simulink model "RTR_IK"  (R2020a)
settings: Solver=ode45  StartTime=0.0  StopTime=T  RelTol=1e-8
values from neighbouring files (symbols this model uses):
  g = 9.81    [TestingIkRTR.m]    (also in TestingScript.m; TestingScriptRTR.m)
  Kd1 = Kp1/10    (= 100)    [TestingIkRTR.m]    (also in TestingScript.m; TestingScriptRTR.m)
  Kp1 = 1000    [TestingIkRTR.m]    (also in TestingScript.m; TestingScriptRTR.m)
  l2 = 0.3    [TestingIkRTR.m]    (also in TestingScriptRTR.m)
  l3 = 0.2    [TestingIkRTR.m]    (also in TestingScriptRTR.m)
  m2 = 20    [TestingIkRTR.m]    (also in TestingScriptRTR.m)
  m3 = 20    [TestingIkRTR.m]    (also in TestingScriptRTR.m)
settings Model: Creator=ja  LastModifiedBy=ja

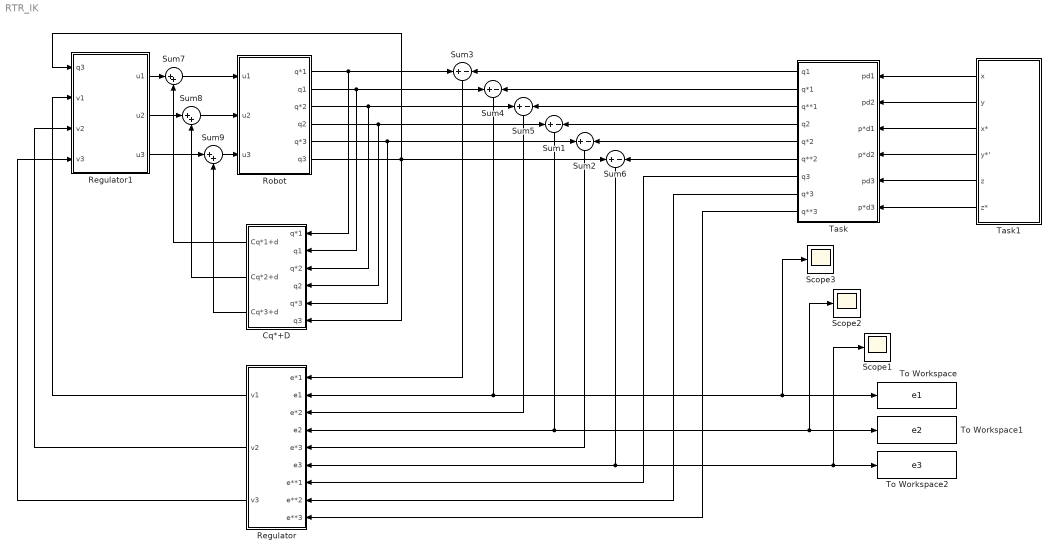
== system RTR_IK ==
  Cq*+D : Subsystem
  Regulator : Subsystem
  Regulator1 : Subsystem
  Robot : Subsystem
  Scope1 : Scope
  Scope2 : Scope
  Scope3 : Scope
  Sum{1..6} (6 alike) : Sum  Inputs=+-
  Sum7 : Sum  Inputs=|++
  Sum8 : Sum  Inputs=|++
  Sum9 : Sum  Inputs=|++
  Task : Subsystem
  Task1 : Subsystem
  To Workspace : ToWorkspace  VariableName=e1  SampleTime=-1
  To Workspace1 : ToWorkspace  VariableName=e2  SampleTime=-1
  To Workspace2 : ToWorkspace  VariableName=e3  SampleTime=-1
  wires:
  Robot/1(q*1) -> Cq*+D/1(q*1), Sum3/1
  Task/1(q1) -> Sum3/2
  Robot/2(q1) -> Cq*+D/2(q1), Sum4/1
  Task/2(q*1) -> Sum4/2
  Task/3(q**1) -> Sum5/2
  Robot/3(q*2) -> Cq*+D/3(q*2), Sum5/1
  Task/4(q2) -> Sum1/2
  Robot/4(q2) -> Cq*+D/4(q2), Sum1/1
  Task/5(q*2) -> Sum2/2
  Robot/5(q*3) -> Cq*+D/5(q*3), Sum2/1
  Task/6(q**2) -> Sum6/2
  Robot/6(q3) -> Regulator1/1(q3), Cq*+D/6(q3), Sum6/1
  Sum3/1 -> Regulator/1(e*1)
  Sum4/1 -> Scope3/1, To Workspace/1, Regulator/2(e1)
  Sum5/1 -> Regulator/3(e*2)
  Sum1/1 -> Scope2/1, To Workspace1/1, Regulator/4(e2)
  Sum2/1 -> Regulator/5(e*3)
  Sum6/1 -> Scope1/1, To Workspace2/1, Regulator/6(e3)
  Regulator/1(" v1") -> Regulator1/2(v1)
  Regulator/2(v2) -> Regulator1/3(v2)
  Regulator/3(v3) -> Regulator1/4(v3)
  Sum7/1 -> Robot/1(u1)
  Regulator1/1(" u1") -> Sum7/1
  Regulator1/2(u2) -> Sum8/1
  Sum8/1 -> Robot/2(u2)
  Regulator1/3(u3) -> Sum9/1
  Sum9/1 -> Robot/3(u3)
  Cq*+D/1(" Cq*1+d") -> Sum7/2
  Cq*+D/2(Cq*2+d) -> Sum8/2
  Cq*+D/3(Cq*3+d) -> Sum9/2
  Task/7(q3) -> Regulator/7(e**1)
  Task/8(q*3) -> Regulator/8(e**2)
  Task/9(q**3) -> Regulator/9(e**3)
  Task1/6(z*) -> Task/6(p*d3)
  Task1/5(z) -> Task/5(pd3)
  Task1/4(y*') -> Task/4(p*d2)
  Task1/1(x) -> Task/1(pd1)
  Task1/2(y) -> Task/2(pd2)
  Task1/3(x*) -> Task/3(p*d1)

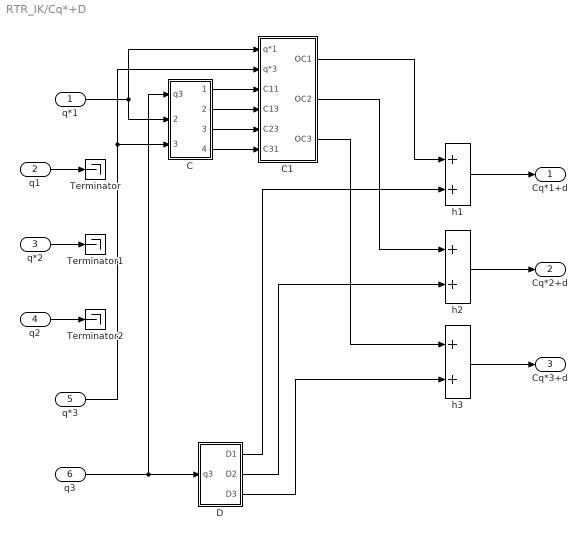
== system RTR_IK/Cq*+D ==
  q*1 : Inport
  q1 : Inport  Port=2
  q*2 : Inport  Port=3
  q2 : Inport  Port=4
  q*3 : Inport  Port=5
  q3 : Inport  Port=6
  C : Subsystem
  C1 : Subsystem
  D : Subsystem
  Terminator : Terminator
  Terminator1 : Terminator
  Terminator2 : Terminator
  h1 : Sum
  h2 : Sum
  h3 : Sum
  " Cq*1+d" : Outport
  Cq*2+d : Outport  Port=2
  Cq*3+d : Outport  Port=3
  wires:
  D/1(D1) -> h1/2
  D/2(D2) -> h2/2
  C1/2(OC2) -> h2/1
  D/3(D3) -> h3/2
  C/2(C13) -> C1/4(C13)
  C/1(C11) -> C1/3(C11)
  C/3(C23) -> C1/5(C23)
  C1/1(OC1) -> h1/1
  C/4(C31) -> C1/6(C31)
  C1/3(OC3) -> h3/1
  q3/1 -> C/1(q3), D/1(q3)
  h1/1 -> " Cq*1+d"/1
  h2/1 -> Cq*2+d/1
  h3/1 -> Cq*3+d/1
  q*1/1 -> C1/1(q*1), C/2(q*1)
  q*3/1 -> C/3(q*3), C1/2(q*3)
  q1/1 -> Terminator/1
  q*2/1 -> Terminator1/1
  q2/1 -> Terminator2/1

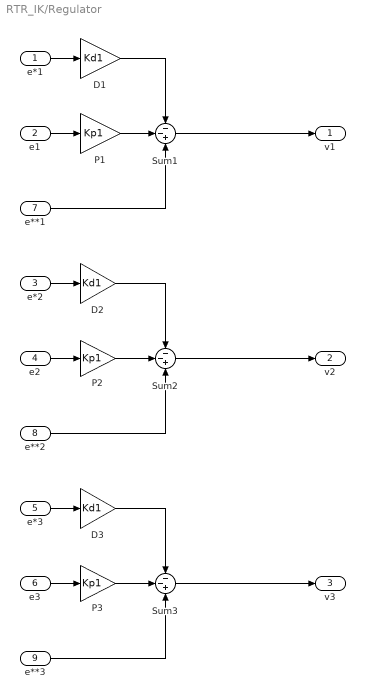
== system RTR_IK/Regulator ==
  e*1 : Inport
  e1 : Inport  Port=2
  e*2 : Inport  Port=3
  e2 : Inport  Port=4
  e*3 : Inport  Port=5
  e3 : Inport  Port=6
  e**1 : Inport  Port=7
  e**2 : Inport  Port=8
  e**3 : Inport  Port=9
  D1 : Gain  Gain=Kd1
  D2 : Gain  Gain=Kd1
  D3 : Gain  Gain=Kd1
  P1 : Gain  Gain=Kp1
  P2 : Gain  Gain=Kp1
  P3 : Gain  Gain=Kp1
  Sum1 : Sum  Inputs=--+
  Sum2 : Sum  Inputs=--+
  Sum3 : Sum  Inputs=--+
  " v1" : Outport
  v2 : Outport  Port=2
  v3 : Outport  Port=3
  wires:
  e2/1 -> P2/1
  Sum2/1 -> v2/1
  e*2/1 -> D2/1
  e1/1 -> P1/1
  Sum1/1 -> " v1"/1
  e*1/1 -> D1/1
  D1/1 -> Sum1/1
  P1/1 -> Sum1/2
  D2/1 -> Sum2/1
  P2/1 -> Sum2/2
  e*3/1 -> D3/1
  Sum3/1 -> v3/1
  P3/1 -> Sum3/2
  D3/1 -> Sum3/1
  e3/1 -> P3/1
  e**1/1 -> Sum1/3
  e**2/1 -> Sum2/3
  e**3/1 -> Sum3/3

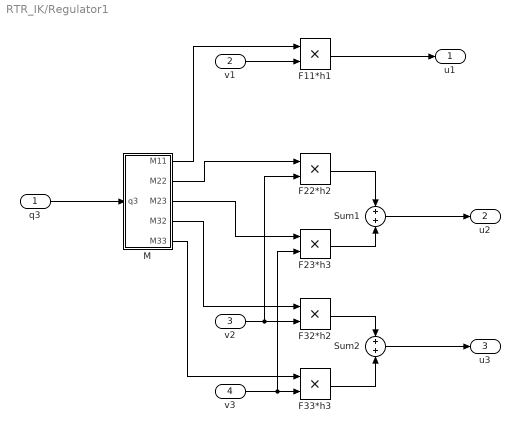
== system RTR_IK/Regulator1 ==
  q3 : Inport
  v1 : Inport  Port=2
  v2 : Inport  Port=3
  v3 : Inport  Port=4
  F11*h1 : Product
  F22*h2 : Product
  F23*h3 : Product
  F32*h2 : Product
  F33*h3 : Product
  M : Subsystem
  Sum1 : Sum
  Sum2 : Sum
  " u1" : Outport
  u2 : Outport  Port=2
  u3 : Outport  Port=3
  wires:
  q3/1 -> M/1(q3)
  F23*h3/1 -> Sum1/2
  F33*h3/1 -> Sum2/2
  F22*h2/1 -> Sum1/1
  F32*h2/1 -> Sum2/1
  v3/1 -> F23*h3/2, F33*h3/2
  v2/1 -> F22*h2/2, F32*h2/2
  v1/1 -> F11*h1/2
  M/1(M11) -> F11*h1/1
  M/2(M22) -> F22*h2/1
  M/3(M23) -> F23*h3/1
  M/4(M32) -> F32*h2/1
  M/5(M33) -> F33*h3/1
  F11*h1/1 -> " u1"/1
  Sum1/1 -> u2/1
  Sum2/1 -> u3/1

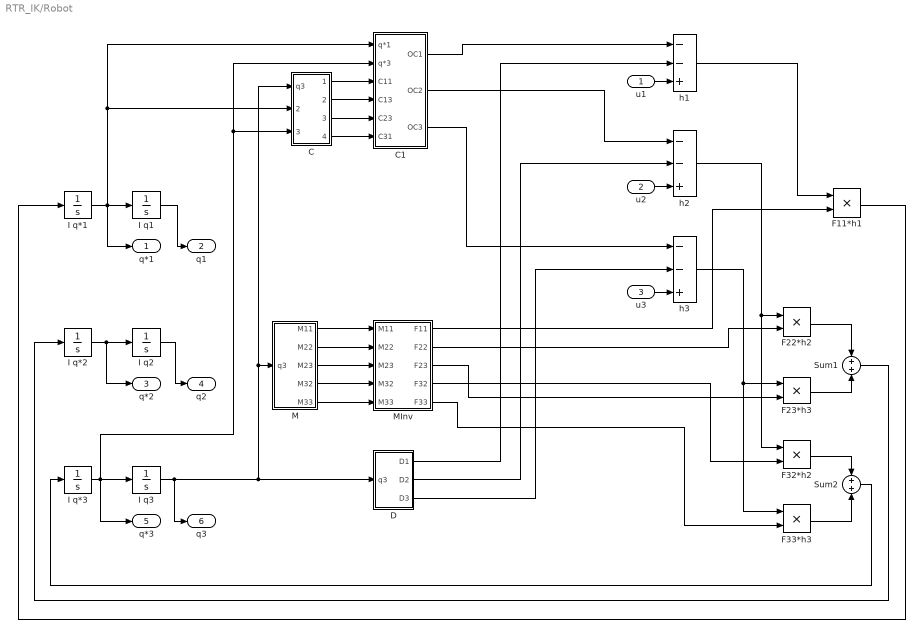
== system RTR_IK/Robot ==
  u1 : Inport
  u2 : Inport  Port=2
  u3 : Inport  Port=3
  C : Subsystem
  C1 : Subsystem
  D : Subsystem
  F11*h1 : Product
  F22*h2 : Product
  F23*h3 : Product
  F32*h2 : Product
  F33*h3 : Product
  I q*1 : Integrator
  I q*2 : Integrator
  I q*3 : Integrator
  I q1 : Integrator
  I q2 : Integrator
  I q3 : Integrator
  M : Subsystem
  MInv : MATLAB Function  TreatAsAtomicUnit=on
  Sum1 : Sum
  Sum2 : Sum
  h1 : Sum  Inputs=--+
  h2 : Sum  Inputs=--+
  h3 : Sum  Inputs=--+
  q*1 : Outport
  q1 : Outport  Port=2
  q*2 : Outport  Port=3
  q2 : Outport  Port=4
  q*3 : Outport  Port=5
  q3 : Outport  Port=6
  wires:
  I q2/1 -> q2/1
  F11*h1/1 -> I q*1/1
  I q*1/1 -> q*1/1, C1/1(q*1), C/2(q*1), I q1/1
  Sum1/1 -> I q*2/1
  I q1/1 -> q1/1
  F23*h3/1 -> Sum1/2
  I q*2/1 -> q*2/1, I q2/1
  F22*h2/1 -> Sum1/1
  u2/1 -> h2/3
  C/1(C11) -> C1/3(C11)
  C/2(C13) -> C1/4(C13)
  C/3(C23) -> C1/5(C23)
  C/4(C31) -> C1/6(C31)
  C1/1(OC1) -> h1/1
  F32*h2/1 -> Sum2/1
  F33*h3/1 -> Sum2/2
  Sum2/1 -> I q*3/1
  I q*3/1 -> C1/2(q*3), C/3(q*3), I q3/1, q*3/1
  I q3/1 -> q3/1, C/1(q3), M/1(q3), D/1(q3)
  u3/1 -> h3/3
  D/3(D3) -> h3/2
  D/2(D2) -> h2/2
  C1/2(OC2) -> h2/1
  C1/3(OC3) -> h3/1
  h2/1 -> F32*h2/1, F22*h2/1
  h3/1 -> F33*h3/1, F23*h3/1
  MInv/2(F22) -> F22*h2/2
  MInv/3(F23) -> F23*h3/2
  MInv/4(F32) -> F32*h2/2
  MInv/5(F33) -> F33*h3/2
  h1/1 -> F11*h1/1
  MInv/1(F11) -> F11*h1/2
  u1/1 -> h1/3
  D/1(D1) -> h1/2
  M/1(M11) -> MInv/1(M11)
  M/2(M22) -> MInv/2(M22)
  M/3(M23) -> MInv/3(M23)
  M/4(M32) -> MInv/4(M32)
  M/5(M33) -> MInv/5(M33)

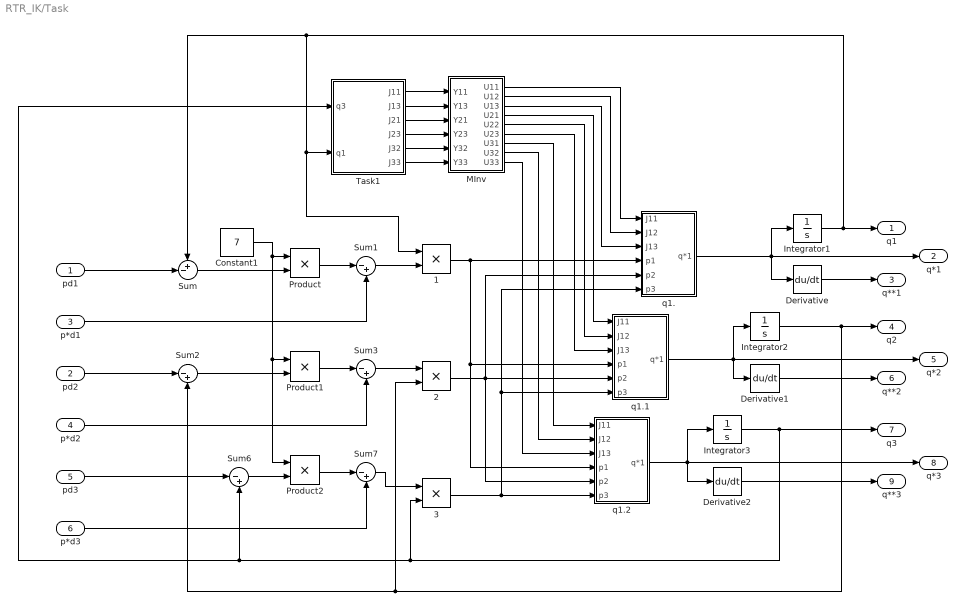
== system RTR_IK/Task ==
  pd1 : Inport
  pd2 : Inport  Port=2
  p*d1 : Inport  Port=3
  p*d2 : Inport  Port=4
  pd3 : Inport  Port=5
  p*d3 : Inport  Port=6
  1 : Product
  2 : Product
  3 : Product
  Constant1 : Constant  Value=7
  Derivative : Derivative
  Derivative1 : Derivative
  Derivative2 : Derivative
  Integrator1 : Integrator
  Integrator2 : Integrator
  Integrator3 : Integrator  InitialCondition=0.1
  MInv : MATLAB Function  TreatAsAtomicUnit=on
  Product : Product
  Product1 : Product
  Product2 : Product
  Sum : Sum  Inputs=+-|
  Sum{1..3,6..7} (5 alike) : Sum  Inputs=|-+
  Task1 : Subsystem
  q1. : Subsystem
  q1.1 : Subsystem
  q1.2 : Subsystem
  q1 : Outport
  q*1 : Outport  Port=2
  q**1 : Outport  Port=3
  q2 : Outport  Port=4
  q*2 : Outport  Port=5
  q**2 : Outport  Port=6
  q3 : Outport  Port=7
  q*3 : Outport  Port=8
  q**3 : Outport  Port=9
  wires:
  pd1/1 -> Sum/2
  Sum1/1 -> 1/2
  Product/1 -> Sum1/1
  Product1/1 -> Sum3/1
  Sum/1 -> Product/2
  Integrator1/1 -> q1/1, Sum/1, 1/1, Task1/2(q1)
  p*d2/1 -> Sum3/2
  Sum2/1 -> Product1/2
  Integrator2/1 -> q2/1, Sum2/2, 2/2
  pd2/1 -> Sum2/1
  p*d1/1 -> Sum1/2
  Sum3/1 -> 2/1
  Sum6/1 -> Product2/2
  pd3/1 -> Sum6/1
  Constant1/1 -> Product2/1, Product1/1, Product/1
  p*d3/1 -> Sum7/2
  Product2/1 -> Sum7/1
  Sum7/1 -> 3/1
  Task1/1(J11) -> MInv/1(Y11)
  Task1/2(J13) -> MInv/2(Y13)
  Task1/3(J21) -> MInv/3(Y21)
  Task1/4(J23) -> MInv/4(Y23)
  Task1/5(J32) -> MInv/5(Y32)
  Task1/6(J33) -> MInv/6(Y33)
  1/1 -> q1./4(p1), q1.2/4(p1), q1.1/4(p1)
  2/1 -> q1.2/5(p2), q1.1/5(p2), q1./5(p2)
  3/1 -> q1./6(p3), q1.1/6(p3), q1.2/6(p3)
  MInv/1(U11) -> q1./1(J11)
  MInv/2(U12) -> q1./2(J12)
  MInv/3(U13) -> q1./3(J13)
  MInv/4(U21) -> q1.1/1(J11)
  MInv/5(U22) -> q1.1/2(J12)
  MInv/6(U23) -> q1.1/3(J13)
  MInv/7(U31) -> q1.2/1(J11)
  MInv/8(U32) -> q1.2/2(J12)
  MInv/9(U33) -> q1.2/3(J13)
  Integrator3/1 -> q3/1, 3/2, Task1/1(q3), Sum6/2
  Derivative/1 -> q**1/1
  q1./1(q*1) -> Derivative/1, Integrator1/1, q*1/1
  q1.1/1(q*1) -> Derivative1/1, Integrator2/1, q*2/1
  q1.2/1(q*1) -> Integrator3/1, Derivative2/1, q*3/1
  Derivative1/1 -> q**2/1
  Derivative2/1 -> q**3/1

== system RTR_IK/Task1 ==
  Clock1 : Clock
  Fcn6 : Fcn  Expr=2*cos(2*u)
  Fcn7 : Fcn  Expr=0.1
  Fcn8 : Fcn  Expr=0.1+u
  Fcn9 : Fcn  Expr=-2*sin(2*u)
  Integrator8 : Integrator
  Integrator9 : Integrator  InitialCondition=1
  x : Outport
  y : Outport  Port=2
  x* : Outport  Port=3
  y*' : Outport  Port=4
  z : Outport  Port=5
  z* : Outport  Port=6
  wires:
  Fcn8/1 -> z/1
  Fcn7/1 -> z*/1
  Integrator8/1 -> x/1
  Fcn6/1 -> x*/1, Integrator8/1
  Clock1/1 -> Fcn8/1, Fcn7/1, Fcn6/1, Fcn9/1
  Integrator9/1 -> y/1
  Fcn9/1 -> y*'/1, Integrator9/1

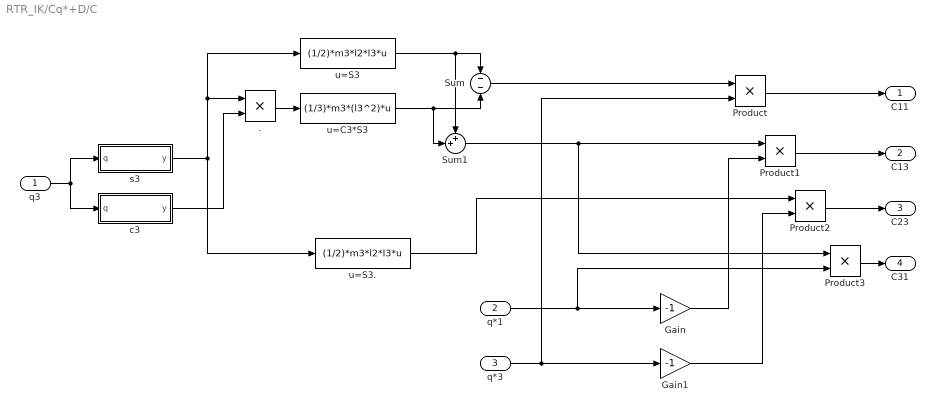
== system RTR_IK/Cq*+D/C ==
  q3 : Inport
  q*1 : Inport  Port=2
  q*3 : Inport  Port=3
  . : Product
  Gain : Gain  Gain=-1
  Gain1 : Gain  Gain=-1
  Product{,1..3} (4 alike) : Product
  Sum : Sum  Inputs=--
  Sum1 : Sum  Inputs=++|
  c3 : MATLAB Function  TreatAsAtomicUnit=on
  s3 : MATLAB Function  TreatAsAtomicUnit=on
  u=C3*S3 : Fcn  Expr=(1/3)*m3*(l3^2)*u
  u=S3 : Fcn  Expr=(1/2)*m3*l2*l3*u
  u=S3. : Fcn  Expr=(1/2)*m3*l2*l3*u
  C11 : Outport
  C13 : Outport  Port=2
  C23 : Outport  Port=3
  C31 : Outport  Port=4
  wires:
  q3/1 -> s3/1(q), c3/1(q)
  c3/1(y) -> ./2
  s3/1(y) -> u=S3./1, ./1, u=S3/1
  ./1 -> u=C3*S3/1
  u=C3*S3/1 -> Sum1/2, Sum/2
  u=S3/1 -> Sum1/1, Sum/1
  Gain1/1 -> Product2/2
  Product/1 -> C11/1
  Product2/1 -> C23/1
  Product1/1 -> C13/1
  Sum/1 -> Product/1
  q*1/1 -> Gain/1, Product3/2
  q*3/1 -> Gain1/1, Product/2
  Product3/1 -> C31/1
  Gain/1 -> Product1/2
  Sum1/1 -> Product1/1, Product3/1
  u=S3./1 -> Product2/1

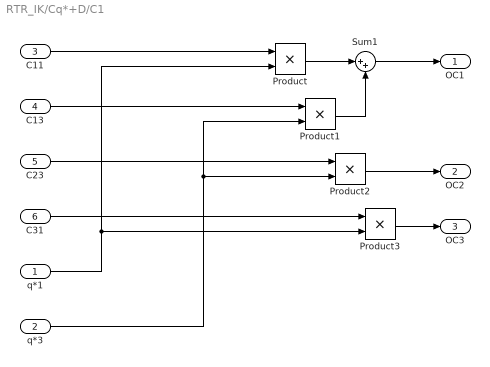
== system RTR_IK/Cq*+D/C1 ==
  q*1 : Inport
  q*3 : Inport  Port=2
  C11 : Inport  Port=3
  C13 : Inport  Port=4
  C23 : Inport  Port=5
  C31 : Inport  Port=6
  Product{,1..3} (4 alike) : Product
  Sum1 : Sum  Inputs=|++
  OC1 : Outport
  OC2 : Outport  Port=2
  OC3 : Outport  Port=3
  wires:
  C11/1 -> Product/1
  C13/1 -> Product1/1
  C23/1 -> Product2/1
  C31/1 -> Product3/1
  Product3/1 -> OC3/1
  Product2/1 -> OC2/1
  q*1/1 -> Product3/2, Product/2
  q*3/1 -> Product2/2, Product1/2
  Product/1 -> Sum1/1
  Sum1/1 -> OC1/1
  Product1/1 -> Sum1/2

== system RTR_IK/Cq*+D/D ==
  q3 : Inport
  . : Fcn  Expr=1/2*m3*l3*u
  Constant : Constant  Value=g
  Constant1 : Constant  Value=m3
  Constant2 : Constant  Value=m2
  Constant3 : Constant  Value=0
  Product : Product
  Product1 : Product
  Sum : Sum
  c3 : MATLAB Function  TreatAsAtomicUnit=on
  D1 : Outport
  D2 : Outport  Port=2
  D3 : Outport  Port=3
  wires:
  c3/1(y) -> ./1
  Sum/1 -> Product/1
  Constant/1 -> Product/2, Product1/1
  ./1 -> Product1/2
  Constant2/1 -> Sum/2
  Constant1/1 -> Sum/1
  q3/1 -> c3/1(q)
  Product/1 -> D2/1
  Product1/1 -> D3/1
  Constant3/1 -> D1/1

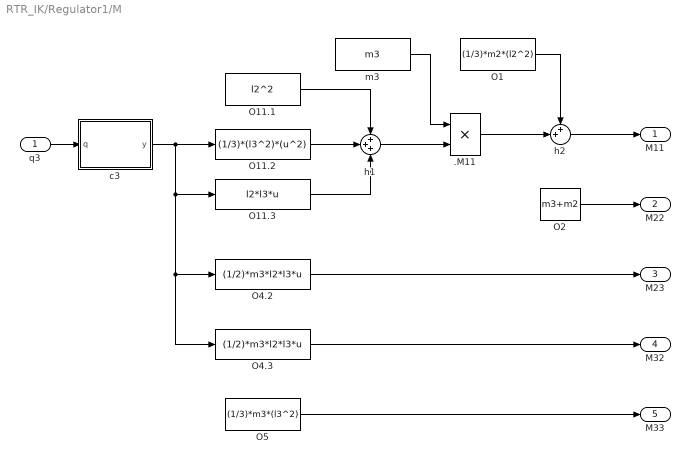
== system RTR_IK/Regulator1/M ==
  q3 : Inport
  .M11 : Product
  O1 : Constant  Value=(1/3)*m2*(l2^2)
  O11.1 : Constant  Value=l2^2
  O11.2 : Fcn  Expr=(1/3)*(l3^2)*(u^2)
  O11.3 : Fcn  Expr=l2*l3*u
  O2 : Constant  Value=m3+m2
  O4.2 : Fcn  Expr=(1/2)*m3*l2*l3*u
  O4.3 : Fcn  Expr=(1/2)*m3*l2*l3*u
  O5 : Constant  Value=(1/3)*m3*(l3^2)
  c3 : MATLAB Function  TreatAsAtomicUnit=on
  h1 : Sum  Inputs=+++
  h2 : Sum  Inputs=++|
  m3 : Constant  Value=m3
  M11 : Outport
  M22 : Outport  Port=2
  M23 : Outport  Port=3
  M32 : Outport  Port=4
  M33 : Outport  Port=5
  wires:
  O1/1 -> h2/1
  O11.3/1 -> h1/3
  m3/1 -> .M11/1
  h1/1 -> .M11/2
  .M11/1 -> h2/2
  O11.1/1 -> h1/1
  O11.2/1 -> h1/2
  h2/1 -> M11/1
  O2/1 -> M22/1
  O4.2/1 -> M23/1
  c3/1(y) -> O11.2/1, O4.3/1, O4.2/1, O11.3/1
  q3/1 -> c3/1(q)
  O5/1 -> M33/1
  O4.3/1 -> M32/1

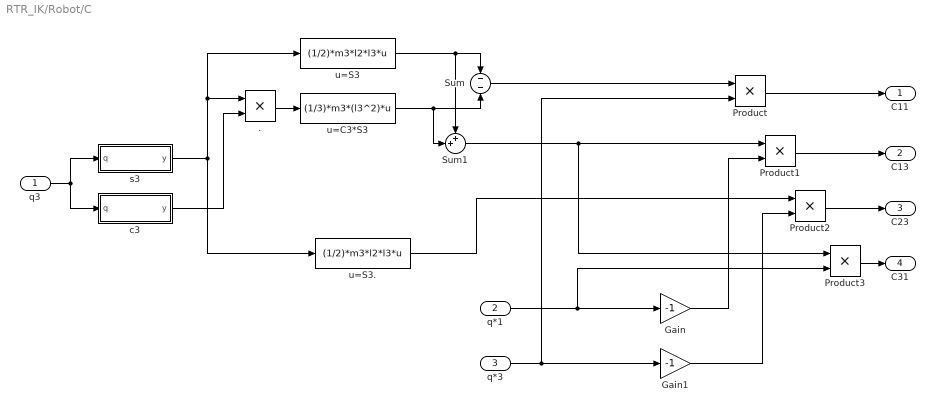
== system RTR_IK/Robot/C ==
  q3 : Inport
  q*1 : Inport  Port=2
  q*3 : Inport  Port=3
  . : Product
  Gain : Gain  Gain=-1
  Gain1 : Gain  Gain=-1
  Product{,1..3} (4 alike) : Product
  Sum : Sum  Inputs=--
  Sum1 : Sum  Inputs=++|
  c3 : MATLAB Function  TreatAsAtomicUnit=on
  s3 : MATLAB Function  TreatAsAtomicUnit=on
  u=C3*S3 : Fcn  Expr=(1/3)*m3*(l3^2)*u
  u=S3 : Fcn  Expr=(1/2)*m3*l2*l3*u
  u=S3. : Fcn  Expr=(1/2)*m3*l2*l3*u
  C11 : Outport
  C13 : Outport  Port=2
  C23 : Outport  Port=3
  C31 : Outport  Port=4
  wires:
  q3/1 -> s3/1(q), c3/1(q)
  c3/1(y) -> ./2
  s3/1(y) -> u=S3./1, ./1, u=S3/1
  ./1 -> u=C3*S3/1
  u=C3*S3/1 -> Sum1/2, Sum/2
  u=S3/1 -> Sum1/1, Sum/1
  Gain1/1 -> Product2/2
  Product/1 -> C11/1
  Product2/1 -> C23/1
  Product1/1 -> C13/1
  Sum/1 -> Product/1
  q*1/1 -> Gain/1, Product3/2
  q*3/1 -> Gain1/1, Product/2
  Product3/1 -> C31/1
  Gain/1 -> Product1/2
  Sum1/1 -> Product1/1, Product3/1
  u=S3./1 -> Product2/1

== system RTR_IK/Robot/C1 ==
  q*1 : Inport
  q*3 : Inport  Port=2
  C11 : Inport  Port=3
  C13 : Inport  Port=4
  C23 : Inport  Port=5
  C31 : Inport  Port=6
  Product{,1..3} (4 alike) : Product
  Sum1 : Sum  Inputs=|++
  OC1 : Outport
  OC2 : Outport  Port=2
  OC3 : Outport  Port=3
  wires:
  C11/1 -> Product/1
  C13/1 -> Product1/1
  C23/1 -> Product2/1
  C31/1 -> Product3/1
  Product3/1 -> OC3/1
  Product2/1 -> OC2/1
  q*1/1 -> Product3/2, Product/2
  q*3/1 -> Product2/2, Product1/2
  Product/1 -> Sum1/1
  Sum1/1 -> OC1/1
  Product1/1 -> Sum1/2

== system RTR_IK/Robot/D ==
  q3 : Inport
  . : Fcn  Expr=1/2*m3*l3*u
  Constant : Constant  Value=g
  Constant1 : Constant  Value=m3
  Constant2 : Constant  Value=m2
  Constant3 : Constant  Value=0
  Product : Product
  Product1 : Product
  Sum : Sum
  c3 : MATLAB Function  TreatAsAtomicUnit=on
  D1 : Outport
  D2 : Outport  Port=2
  D3 : Outport  Port=3
  wires:
  c3/1(y) -> ./1
  Sum/1 -> Product/1
  Constant/1 -> Product/2, Product1/1
  ./1 -> Product1/2
  Constant2/1 -> Sum/2
  Constant1/1 -> Sum/1
  q3/1 -> c3/1(q)
  Product/1 -> D2/1
  Product1/1 -> D3/1
  Constant3/1 -> D1/1

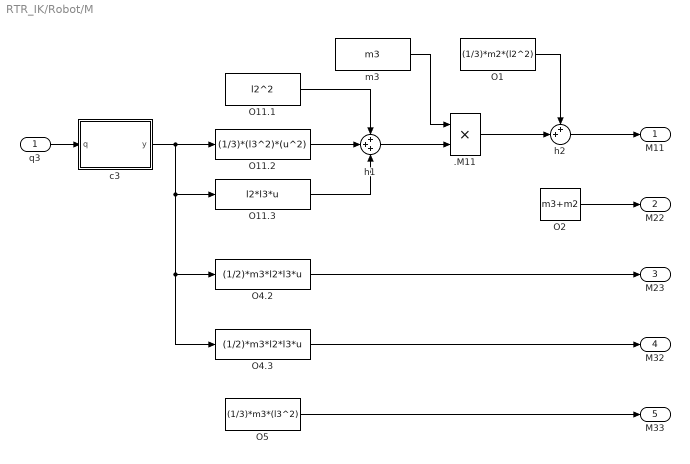
== system RTR_IK/Robot/M ==
  q3 : Inport
  .M11 : Product
  O1 : Constant  Value=(1/3)*m2*(l2^2)
  O11.1 : Constant  Value=l2^2
  O11.2 : Fcn  Expr=(1/3)*(l3^2)*(u^2)
  O11.3 : Fcn  Expr=l2*l3*u
  O2 : Constant  Value=m3+m2
  O4.2 : Fcn  Expr=(1/2)*m3*l2*l3*u
  O4.3 : Fcn  Expr=(1/2)*m3*l2*l3*u
  O5 : Constant  Value=(1/3)*m3*(l3^2)
  c3 : MATLAB Function  TreatAsAtomicUnit=on
  h1 : Sum  Inputs=+++
  h2 : Sum  Inputs=++|
  m3 : Constant  Value=m3
  M11 : Outport
  M22 : Outport  Port=2
  M23 : Outport  Port=3
  M32 : Outport  Port=4
  M33 : Outport  Port=5
  wires:
  O1/1 -> h2/1
  O11.3/1 -> h1/3
  m3/1 -> .M11/1
  h1/1 -> .M11/2
  .M11/1 -> h2/2
  O11.1/1 -> h1/1
  O11.2/1 -> h1/2
  h2/1 -> M11/1
  O2/1 -> M22/1
  O4.2/1 -> M23/1
  c3/1(y) -> O11.2/1, O4.3/1, O4.2/1, O11.3/1
  q3/1 -> c3/1(q)
  O5/1 -> M33/1
  O4.3/1 -> M32/1

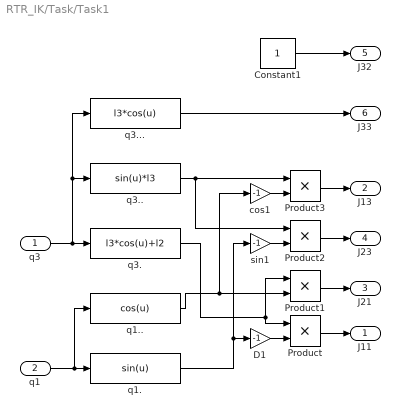
== system RTR_IK/Task/Task1 ==
  q3 : Inport
  q1 : Inport  Port=2
  Constant1 : Constant
  D1 : Gain  Gain=-1
  Product{,1..3} (4 alike) : Product
  cos1 : Gain  Gain=-1
  q1. : Fcn  Expr=sin(u)
  q1.. : Fcn  Expr=cos(u)
  q3. : Fcn  Expr=l3*cos(u)+l2
  q3.. : Fcn  Expr=sin(u)*l3
  q3... : Fcn  Expr=l3*cos(u)
  sin1 : Gain  Gain=-1
  J11 : Outport
  J13 : Outport  Port=2
  J21 : Outport  Port=3
  J23 : Outport  Port=4
  J32 : Outport  Port=5
  J33 : Outport  Port=6
  wires:
  q3/1 -> q3.../1, q3../1, q3./1
  q1/1 -> q1../1, q1./1
  q3./1 -> Product/1, Product1/1
  Product/1 -> J11/1
  D1/1 -> Product/2
  q1./1 -> sin1/1, D1/1
  q1../1 -> cos1/1, Product1/2
  q3../1 -> Product2/1, Product3/1
  sin1/1 -> Product2/2
  cos1/1 -> Product3/2
  Product3/1 -> J13/1
  Product1/1 -> J21/1
  Product2/1 -> J23/1
  q3.../1 -> J33/1
  Constant1/1 -> J32/1

== system RTR_IK/Task/q1. ==
  J11 : Inport
  J12 : Inport  Port=2
  J13 : Inport  Port=3
  p1 : Inport  Port=4
  p2 : Inport  Port=5
  p3 : Inport  Port=6
  J1*q1 : Product
  J2*q2 : Product
  J3*q3 : Product
  Sum8 : Sum  Inputs=+++
  q*1 : Outport
  wires:
  J11/1 -> J1*q1/1
  p1/1 -> J1*q1/2
  J12/1 -> J2*q2/1
  J13/1 -> J3*q3/1
  p2/1 -> J2*q2/2
  p3/1 -> J3*q3/2
  J2*q2/1 -> Sum8/2
  J1*q1/1 -> Sum8/1
  J3*q3/1 -> Sum8/3
  Sum8/1 -> q*1/1

== system RTR_IK/Task/q1.1 ==
  J11 : Inport
  J12 : Inport  Port=2
  J13 : Inport  Port=3
  p1 : Inport  Port=4
  p2 : Inport  Port=5
  p3 : Inport  Port=6
  J1*q1 : Product
  J2*q2 : Product
  J3*q3 : Product
  Sum8 : Sum  Inputs=+++
  q*1 : Outport
  wires:
  J11/1 -> J1*q1/1
  p1/1 -> J1*q1/2
  J12/1 -> J2*q2/1
  J13/1 -> J3*q3/1
  p2/1 -> J2*q2/2
  p3/1 -> J3*q3/2
  J2*q2/1 -> Sum8/2
  J1*q1/1 -> Sum8/1
  J3*q3/1 -> Sum8/3
  Sum8/1 -> q*1/1

== system RTR_IK/Task/q1.2 ==
  J11 : Inport
  J12 : Inport  Port=2
  J13 : Inport  Port=3
  p1 : Inport  Port=4
  p2 : Inport  Port=5
  p3 : Inport  Port=6
  J1*q1 : Product
  J2*q2 : Product
  J3*q3 : Product
  Sum8 : Sum  Inputs=+++
  q*1 : Outport
  wires:
  J11/1 -> J1*q1/1
  p1/1 -> J1*q1/2
  J12/1 -> J2*q2/1
  J13/1 -> J3*q3/1
  p2/1 -> J2*q2/2
  p3/1 -> J3*q3/2
  J2*q2/1 -> Sum8/2
  J1*q1/1 -> Sum8/1
  J3*q3/1 -> Sum8/3
  Sum8/1 -> q*1/1

== matlab function RTR_IK/Robot/M/c3 ==
  data: q input; y output
function y = c(q)

y = cos(q);

== matlab function RTR_IK/Robot/C/c3 ==
  data: q input; y output
function y = c(q)

y = cos(q);

== matlab function RTR_IK/Robot/D/c3 ==
  data: q input; y output
function y = c(q)

y = cos(q);

== matlab function RTR_IK/Cq*+D/C/c3 ==
  data: q input; y output
function y = c(q)

y = cos(q);

== matlab function RTR_IK/Robot/C/s3 ==
  data: q input; y output
function y = s(q)

y = sin(q);

== matlab function RTR_IK/Robot/MInv ==
  data: M11 input; M22 input; F11 output; F22 output; M23 input; M32 input; F23 output; F32 output; M33 input; F33 output
function [F11, F22, F23, F32, F33] = c(M11, M22, M23, M32, M33)

M = [M11 0 0; 0 M22 M23; 0 M32 M33];
F = inv(M);

F11 = F(1);
F22 = F(5);
F23 = F(6);
F32 = F(8);
F33 = F(9);

== matlab function RTR_IK/Cq*+D/C/s3 ==
  data: q input; y output
function y = s(q)

y = sin(q);

== matlab function RTR_IK/Cq*+D/D/c3 ==
  data: q input; y output
function y = c(q)

y = cos(q);

== matlab function RTR_IK/Regulator1/M/c3 ==
  data: q input; y output
function y = c(q)

y = cos(q);

== matlab function RTR_IK/Task/MInv ==
  data: Y11 input; Y13 input; Y21 input; Y23 input; Y32 input; U11 output; U12 output; U13 output; Y33 input; U21 output; U22 output; U23 output; U31 output; U32 output; U33 output
function [U11, U12, U13, U21, U22, U23, U31, U32, U33] = c(Y11, Y13, Y21, Y23, Y32, Y33)

M = [Y11 0 Y13; Y21 0 Y23; 0 Y32 Y33];
F = inv(M);

U11 = F(1);
U12 = F(2);
U13 = F(3);
U21 = F(4);
U22 = F(5);
U23 = F(6);
U31 = F(7);
U32 = F(9);
U33 = F(9);
